simulink model "SNN"  (R2025b)
settings: Solver=VariableStepAuto  StartTime=0.0  StopTime=0.064  RelTol=1e-3
settings Model: Creator=madew  LastModifiedBy=madew

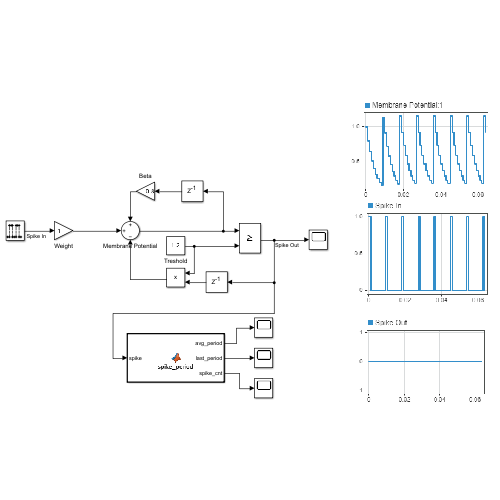
[thumbnail: Simulink's stored preview of the top-level diagram]
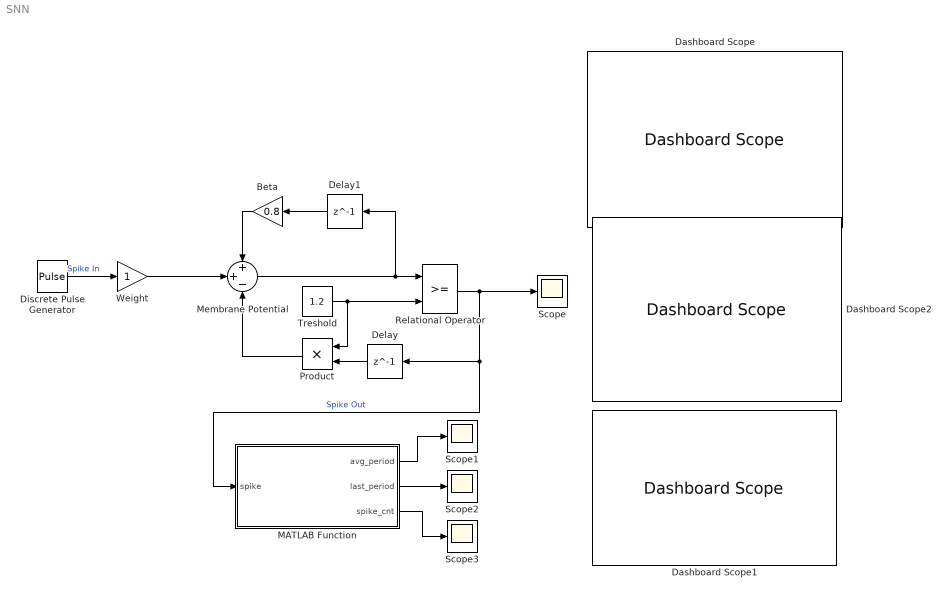
== system SNN ==
  Beta : Gain  Gain=0.8
  Dashboard Scope : DashboardScope  FontColor=[0.0, 0.0, 0.0]
  Dashboard Scope1 : DashboardScope  FontColor=[0.0, 0.0, 0.0]
  Dashboard Scope2 : DashboardScope  FontColor=[0.0, 0.0, 0.0]
  Delay : Delay  DelayLength=1  InitialCondition=0
  Delay1 : Delay  DelayLength=1  InitialCondition=0
  Discrete Pulse Generator : DiscretePulseGenerator  Period=9  SampleTime=0.001
  MATLAB Function : MATLAB Function  TreatAsAtomicUnit=on
  Membrane Potential : Sum  Inputs=++-
  Product : Product
  Relational Operator : RelationalOperator  OutDataTypeStr=boolean  RndMeth=Simplest  InputSameDT=off
  Scope{,1..3} (4 alike) : Scope
      Scope settings: ActiveDisplayYMinimum=-1  ActiveDisplayYMaximum=1
      Scope1 settings: ActiveDisplayYMinimum=-0.00031864342060336916  ActiveDisplayYMaximum=0.001166629247756003
      Scope2 settings: ActiveDisplayYMinimum=0.0019190130258828081  ActiveDisplayYMaximum=0.00351710145886039  DataLoggingVariableName=ScopeData2
      Scope3 settings: ActiveDisplayYMinimum=-1  ActiveDisplayYMaximum=1  DataLoggingVariableName=ScopeData3
  Treshold : Constant  Value=1.2
  Weight : Gain
  wires:
  Delay1/1 -> Beta/1
  Beta/1 -> Membrane Potential/1
  Delay/1 -> Product/2
  Treshold/1 -> Product/1, Relational Operator/2
  Product/1 -> Membrane Potential/3
  Membrane Potential/1 -> Delay1/1, Relational Operator/1
  Relational Operator/1 -> Scope/1, MATLAB Function/1(spike), Delay/1  "Spike Out"
  Weight/1 -> Membrane Potential/2
  MATLAB Function/1(avg_period) -> Scope1/1
  MATLAB Function/2(last_period) -> Scope2/1
  MATLAB Function/3(spike_cnt) -> Scope3/1
  Discrete Pulse Generator/1 -> Weight/1  "Spike In"

== matlab function SNN/MATLAB Function ==
  data: spike input; avg_period output; last_period output; spike_cnt output
function [avg_period, last_period, spike_cnt] = spike_period(spike)
%#codegen
% spike     : input logika (boolean) 0/1
% avg_period: rata-rata periode antar spike (detik)
% last_period: periode spike terakhir (detik)
% spike_cnt : jumlah spike yang sudah terjadi

persistent prev_spike last_time total_time spike_cnt_int Ts t

if isempty(prev_spike)
    % Semua persistent diset dengan tipe konsisten
    prev_spike   = false;   % LOGICAL, bukan 0
    last_time    = 0.0;     % DOUBLE
    total_time   = 0.0;     % DOUBLE
    spike_cnt_int = 0.0;    % DOUBLE (counter)
    Ts           = 1e-4;    % SAMPLE TIME (detik) -> ganti sesuai model kamu
    t            = 0.0;     % waktu sekarang (DOUBLE)
end

% Naikkan waktu
t = t + Ts;

% Default output
last_period = 0.0;
avg_period  = 0.0;

% Deteksi rising edge: 0 -> 1
if spike && ~prev_spike
    if spike_cnt_int > 0
        % Hitung periode (detik) = selisih waktu antar spike
        last_period = t - last_time;
        total_time  = total_time + last_period;
    end
    
    last_time     = t;
    spike_cnt_int = spike_cnt_int + 1.0;
end

% Hitung rata-rata periode (hanya jika sudah ada >= 2 spike)
if spike_cnt_int > 1.0
    avg_period = total_time / (spike_cnt_int - 1.0);
else
    avg_period = 0.0;
end

% Simpan spike sekarang sebagai previous utk sample berikutnya
prev_spike = spike;

% Output jumlah spike
spike_cnt = spike_cnt_int;
